simulink model "test_margin_Angle_control_loop"  (Simulink 7.8)
settings: Solver=ode4  StartTime=0.0  StopTime=2  FixedStep=0.005  RelTol=1e-3
values from neighbouring files (symbols this model uses):
  Kd_omega = ( 2*Z_omega*W_omega + r_omega - 2*Zm*Wm ) / (Km*Wm^2)    [Automatic_Control.m]
  Ki_omega = r_omega*W_omega^2 / (Km*Wm^2)    [Automatic_Control.m]
  Km = num_motor(3) / den_motor(3)    [Automatic_Control.m]    (also in Gimbal_Motor_Modeling.m = (num_m(3))/den_m(3))
  Kp_omega = ( 2*Z_omega*W_omega*r_omega + W_omega^2 - Wm^2) / (Km*Wm^2)    [Automatic_Control.m]
  Kt_angle = W_angle^2 / Tm    [Automatic_Control.m]
  Kw_angle = (2*Z_angle*W_angle - Tm ) / Tm    [Automatic_Control.m]
  tau = 4*Z_omega*W_omega    (= 96)    [Automatic_Control.m]
  Wm = den_motor(3)^0.5    [Automatic_Control.m]    (also in Gimbal_Motor_Modeling.m = (den_m(3))^0.5)
  Zm = den_motor(2) / 2 / Wm    [Automatic_Control.m]    (also in Gimbal_Motor_Modeling.m = (den_m(2)) / 2 / Wm)
settings Model: Creator=mechatronics  LastModifiedBy=mechatronics  BufferReuse=off
settings OptimizationCC: InlineParams=on  BufferReuse=off
settings DebuggingCC: InitInArrayFormatMsg=none

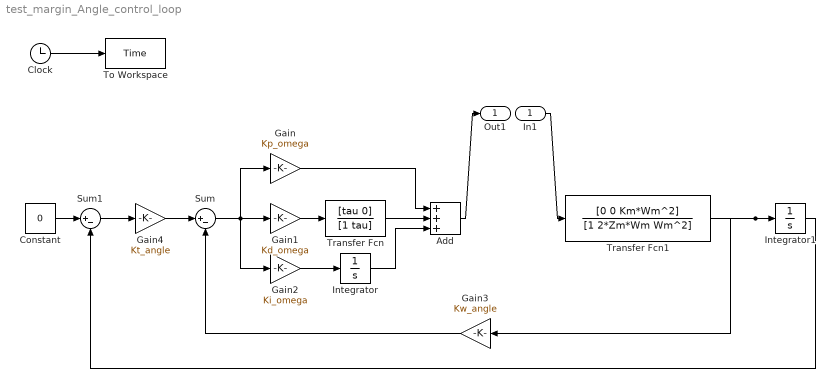
== system test_margin_Angle_control_loop ==
  In1 : Inport
  Add : Sum  Inputs=+++
  Clock : Clock
  Constant : Constant  Value=0
  Gain : Gain  Gain=Kp_omega
  Gain1 : Gain  Gain=Kd_omega
  Gain2 : Gain  Gain=Ki_omega
  Gain3 : Gain  Gain=Kw_angle
  Gain4 : Gain  Gain=Kt_angle
  Integrator : Integrator
  Integrator1 : Integrator
  Sum : Sum  Inputs=|+-
  Sum1 : Sum  Inputs=|+-
  To Workspace : ToWorkspace  VariableName=Time  SampleTime=-1  SaveFormat=Array
  Transfer Fcn : TransferFcn  Numerator=[tau 0]  Denominator=[1 tau]
  Transfer Fcn1 : TransferFcn  Numerator=[0 0 Km*Wm^2]  Denominator=[1 2*Zm*Wm Wm^2]
  Out1 : Outport
  wires:
  Clock/1 -> To Workspace/1
  Gain2/1 -> Integrator/1
  Gain1/1 -> Transfer Fcn/1
  Sum/1 -> Gain1/1, Gain/1, Gain2/1
  Gain/1 -> Add/1
  Transfer Fcn/1 -> Add/2
  Integrator/1 -> Add/3
  Gain4/1 -> Sum/1
  Transfer Fcn1/1 -> Integrator1/1, Gain3/1
  Integrator1/1 -> Sum1/2
  Sum1/1 -> Gain4/1
  Gain3/1 -> Sum/2
  Constant/1 -> Sum1/1
  In1/1 -> Transfer Fcn1/1
  Add/1 -> Out1/1
